simulink model "My_Nonlinear_with_controller"  (R2021b)
settings: Solver=VariableStepAuto  StartTime=0.0  StopTime=simTime  RelTol=1e-3
undefined symbols (not defined in the file): b, D, g, k, L, m, MoI, omega, p, p_dot, RPM, set_point, TakeStep, Theta
libraries: slpidlib x2
settings Model: Creator=Wojciech  LastModifiedBy=tanzc

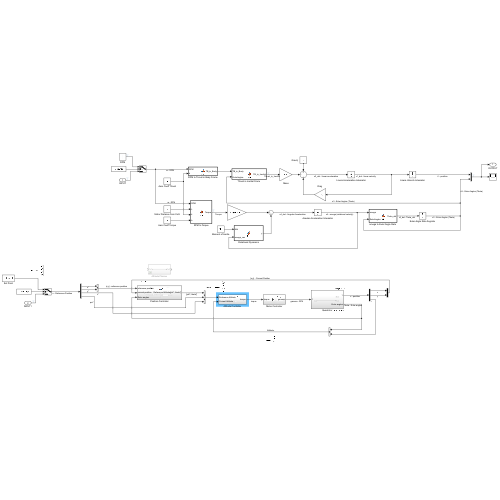
[thumbnail: Simulink's stored preview of the top-level diagram]
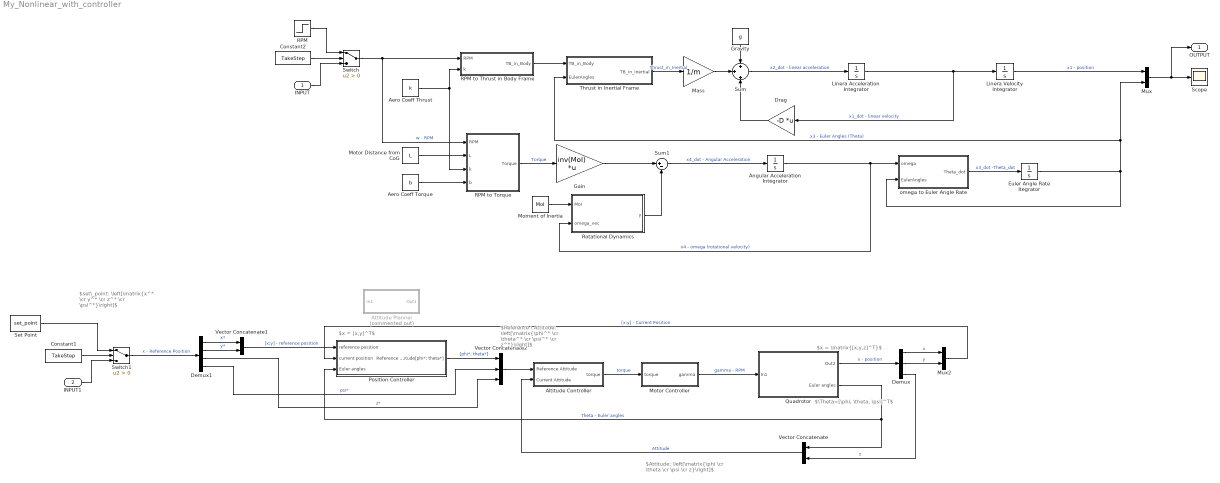
== system My_Nonlinear_with_controller ==
  note: $x = [x,y]^T$
  note: $\Theta=[\phi, \theta, \psi]^T$
  note: $x = \matrix{[x,y,z]^T}$
  note: $Attitude: \left[\matrix{\phi \cr \theta \cr \psi \cr z}\right]$
  note: $set\_point: \left[\matrix{x^* \cr y^* \cr z^* \cr \psi^*}\right]$
  note: $Reference \ Attitude: \left[\matrix{\phi^* \cr \theta^* \cr \psi^* \cr z^*}\right]$
  INPUT : Inport  PortDimensions=4
  INPUT1 : Inport  Port=2  PortDimensions=4
  Aero Coeff Thrust : Constant  Value=k
  Aero Coeff Torque : Constant  Value=b
  Altitude Controller : Subsystem
  Angular Acceleration Integrator : Integrator  Priority=4  InitialCondition=omega
  Attitude Planner : Subsystem  Commented=on
  Constant1 : Constant  Value=TakeStep
  Constant2 : Constant  Value=TakeStep
  Demux : Demux  Outputs=3
  Demux1 : Demux
  Drag : Gain  Gain=-D  Multiplication=Matrix(K*u)
  Euler Angle Rate Itegrator : Integrator  Priority=3  InitialCondition=Theta
  Gain : Gain  Gain=inv(MoI)  Multiplication=Matrix(K*u)
  Gravity : Constant  Value=g  VectorParams1D=off
  Linera Acceleration Integrator : Integrator  Priority=2  InitialCondition=p_dot
  Linera Velocity Integrator : Integrator  Priority=1  InitialCondition=p
  Mass : Gain  Gain=1/m
  Moment of Inertia : Constant  Value=MoI  VectorParams1D=off
  Motor Controller : Subsystem
  Motor Distance from CoG : Constant  Value=L
  Mux : Mux  Inputs=2
  Mux2 : Mux  Inputs=2
  Position Controller : Subsystem
  Quadrotor : Subsystem
  RPM : Step  Time=0  After=RPM  SampleTime=0
  RPM to Thrust in Body Frame : MATLAB Function  TreatAsAtomicUnit=on
  RPM to Torque : MATLAB Function  TreatAsAtomicUnit=on
  Rotational Dynamics : MATLAB Function  TreatAsAtomicUnit=on
  Scope : Scope
  Set Point : Constant  Value=set_point
  Sum : Sum  Inputs=+|+|+
  Sum1 : Sum  Inputs=|+-
  Switch : Switch  Criteria=u2 > Threshold
  Switch1 : Switch  Criteria=u2 > Threshold
  Thrust in Inertial Frame : MATLAB Function  TreatAsAtomicUnit=on
  Vector Concatenate : Concatenate
  Vector Concatenate1 : Concatenate
  Vector Concatenate2 : Concatenate  NumInputs=3
  "omega to Euler Angle Rate " : MATLAB Function  TreatAsAtomicUnit=on
  OUTPUT : Outport
  wires:
  Linera Velocity Integrator/1 -> Mux/1  "x1 - position"
  Linera Acceleration Integrator/1 -> Drag/1, Linera Velocity Integrator/1  "x1_dot - linear velocity"
  Sum/1 -> Linera Acceleration Integrator/1  "x2_dot - linear acceleration"
  Gravity/1 -> Sum/1
  RPM to Thrust in Body Frame/1(TB_in_Body) -> Thrust in Inertial Frame/1(TB_in_Body)
  Aero Coeff Thrust/1 -> RPM to Thrust in Body Frame/2(k), RPM to Torque/3(k)
  Thrust in Inertial Frame/1(TB_in_Inertial) -> Mass/1  "Thrust_in_Inertial"
  Mass/1 -> Sum/2
  Drag/1 -> Sum/3
  Motor Distance from CoG/1 -> RPM to Torque/2(L)
  Aero Coeff Torque/1 -> RPM to Torque/4(b)
  RPM to Torque/1(Torque) -> Gain/1  "Torque"
  Gain/1 -> Sum1/1
  Rotational Dynamics/1(y) -> Sum1/2
  Moment of Inertia/1 -> Rotational Dynamics/1(MoI)
  Sum1/1 -> Angular Acceleration Integrator/1  "x4_dot - Angular Acceleration"
  Angular Acceleration Integrator/1 -> "omega to Euler Angle Rate "/1(omega), Rotational Dynamics/2(omega_vec)  "x4 - omega (rotational velocity)"
  "omega to Euler Angle Rate "/1(Theta_dot) -> Euler Angle Rate Itegrator/1  "x3_dot -Theta_dot"
  Euler Angle Rate Itegrator/1 -> Mux/2, Thrust in Inertial Frame/2(EulerAngles), "omega to Euler Angle Rate "/2(EulerAngles)  "x3 - Euler Angles (Theta)"
  Mux/1 -> OUTPUT/1, Scope/1
  Constant2/1 -> Switch/2
  INPUT/1 -> Switch/3
  RPM/1 -> Switch/1
  Switch/1 -> RPM to Thrust in Body Frame/1(RPM), RPM to Torque/1(RPM)  "w - RPM"
  Quadrotor/1(Out2) -> Demux/1  "x - position"
  Quadrotor/2(Euler angles) -> Position Controller/3(Euler angles), Vector Concatenate/1  "Theta - Euler angles"
  Vector Concatenate/1 -> Altitude Controller/2(Current Attitude)  "Attitude"
  Demux/1 -> Mux2/1  "x"
  Demux/2 -> Mux2/2  "y"
  Mux2/1 -> Position Controller/2(current position)  "[x;y] - Current Position"
  Set Point/1 -> Switch1/1
  Constant1/1 -> Switch1/2
  INPUT1/1 -> Switch1/3
  Motor Controller/1(gamma) -> Quadrotor/1(In1)  "gamma - RPM"
  Altitude Controller/1(torque) -> Motor Controller/1(torque)  "torque"
  Switch1/1 -> Demux1/1  "x - Reference Position"
  Demux1/1 -> Vector Concatenate1/1  "x*"
  Demux1/2 -> Vector Concatenate1/2  "y*"
  Demux1/3 -> Vector Concatenate2/3  "z*"
  Vector Concatenate1/1 -> Position Controller/1(reference position)  "[x;y] - reference position"
  Position Controller/1(Reference Attitude[phi*; theta*]) -> Vector Concatenate2/1  "[phi*; theta*]"
  Vector Concatenate2/1 -> Altitude Controller/1(Reference Attitude)
  Demux1/4 -> Vector Concatenate2/2  "psi*"
  Demux/3 -> Vector Concatenate/2  "z"

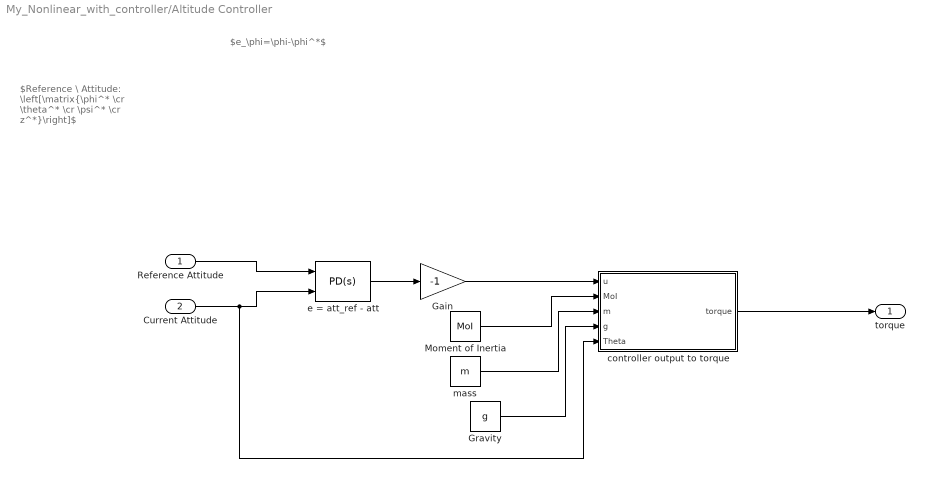
== system My_Nonlinear_with_controller/Altitude Controller ==
  note: $e_\phi=\phi-\phi^*$
  note: $Reference \ Attitude: \left[\matrix{\phi^* \cr \theta^* \cr \psi^* \cr z^*}\right]$
  Reference Attitude : Inport
  Current Attitude : Inport  Port=2
  Gain : Gain  Gain=-1
  Gravity : Constant  Value=g  VectorParams1D=off
  Moment of Inertia : Constant  Value=MoI  VectorParams1D=off
  controller output to torque : MATLAB Function  TreatAsAtomicUnit=on
  e = att_ref - att : slpidlib/PID Controller (2DOF)  Controller=PD  Form=Parallel  TimeDomain=Continuous-time  UseExternalTs=off  SampleTime=-1  IntegratorMethod=Forward Euler  FilterMethod=Forward Euler  ControllerParametersSource=internal  P=1  I=1  D=0  UseFilter=on  N=100  b=1  c=1  TunerSelectOption=Transfer Function Based (PID Tuner App)  InitialConditionSource=internal  InitialConditionForIntegrator=0  InitialConditionForFilter=0  DifferentiatorICPrevScaledInput=0  ExternalReset=none  TrackingMode=off  Kt=1  LimitOutput=off  SatLimitsSource=internal  UpperSaturationLimit=inf  LowerSaturationLimit=-inf  LinearizeAsGain=on  AntiWindupMode=none  Kb=1  POutMin=[]  POutMax=[]  IOutMin=[]  IOutMax=[]  DOutMin=[]  DOutMax=[]  NOutMin=[]  NOutMax=[]  bOutMin=[]  bOutMax=[]  cOutMin=[]  cOutMax=[]  SumOutMin=[]  SumOutMax=[]  SaturationOutMin=[]  SaturationOutMax=[]  PParamMin=[]  PParamMax=[]  IParamMin=[]  IParamMax=[]  DParamMin=[]  DParamMax=[]  NParamMin=[]  NParamMax=[]  bParamMin=[]  bParamMax=[]  cParamMin=[]  cParamMax=[]  KbParamMin=[]  KbParamMax=[]  KtParamMin=[]  KtParamMax=[]  KbOutMin=[]  KbOutMax=[]  KtOutMin=[]  KtOutMax=[]  IntegratorOutMin=[]  IntegratorOutMax=[]  FilterOutMin=[]  FilterOutMax=[]  SumI1OutMin=[]  SumI1OutMax=[]  SumI2OutMin=[]  SumI2OutMax=[]  SumI3OutMin=[]  SumI3OutMax=[]  SumI4OutMin=[]  SumI4OutMax=[]  SumDOutMin=[]  SumDOutMax=[]  Sum1OutMin=[]  Sum1OutMax=[]  Sum2OutMin=[]  Sum2OutMax=[]  Sum3OutMin=[]  Sum3OutMax=[]  DifferentiatorOutMin=[]  DifferentiatorOutMax=[]  FilterDiffOutCoefMin=[]  FilterDiffOutCoefMax=[]  ReciprocalOutMin=[]  ReciprocalOutMax=[]  SumDenOutMin=[]  SumDenOutMax=[]  SumNumOutMin=[]  SumNumOutMax=[]  DivideOutMin=[]  DivideOutMax=[]  UdiffTsProdOutMin=[]  UdiffTsProdOutMax=[]  NTsProdOutMin=[]  NTsProdOutMax=[]  UintegralTsProdOutMin=[]  UintegralTsProdOutMax=[]  UngainTsProdOutMin=[]  UngainTsProdOutMax=[]  IntegratorContinuousStateAttributes=''  IntegratorStateMustResolveToSignalObject=off  IntegratorRTWStateStorageClass=Auto  FilterContinuousStateAttributes=''  FilterStateMustResolveToSignalObject=off  FilterRTWStateStorageClass=Auto  ParallelPVariant=InternalParameters  IdealPVariant=Disabled  IVariant=Disabled  DVariant=InternalParameters  bVariant=InternalParameters  cVariant=InternalParameters  IntegratorVariant=Disabled  SatVariant=Disabled  AWVariant=Disabled  PCopyVariant=Disabled  TRVariant=Disabled  FdbkBlocksVariant=Forward  IdealPFdbkVariant=Disabled  SatFdbkVariant=Disabled  DerivativeFilterVariant=ContFilter  NVariant=InternalParameters  NCopyVariant=Disabled  FilterICVariant=InternalICsFilter  IntegratorICVariant=Disabled  ExternalResetVariant=Disabled  TRSumVariant=Passthrough  SumFdbkVariant=Disabled  SumVariant=Sum_PD  TsampFilterVariant=InternalTs  TsampNgainVariant=Passthrough  TsampIntegralVariant=Disabled_SignalSpec  ExternalSaturationOutDataTypeStr=Inherit: Same as second input
      settings: SourceProductBaseCode=SL
  mass : Constant  Value=m
  torque : Outport
  wires:
  Reference Attitude/1 -> e = att_ref - att/1
  Current Attitude/1 -> controller output to torque/5(Theta), e = att_ref - att/2
  e = att_ref - att/1 -> Gain/1
  Gain/1 -> controller output to torque/1(u)
  Moment of Inertia/1 -> controller output to torque/2(MoI)
  mass/1 -> controller output to torque/3(m)
  Gravity/1 -> controller output to torque/4(g)
  controller output to torque/1(torque) -> torque/1

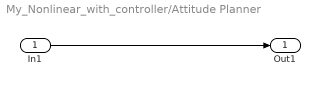
== system My_Nonlinear_with_controller/Attitude Planner ==
  In1 : Inport
  Out1 : Outport
  wires:
  In1/1 -> Out1/1

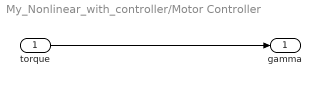
== system My_Nonlinear_with_controller/Motor Controller ==
  torque : Inport
  gamma : Outport
  wires:
  torque/1 -> gamma/1

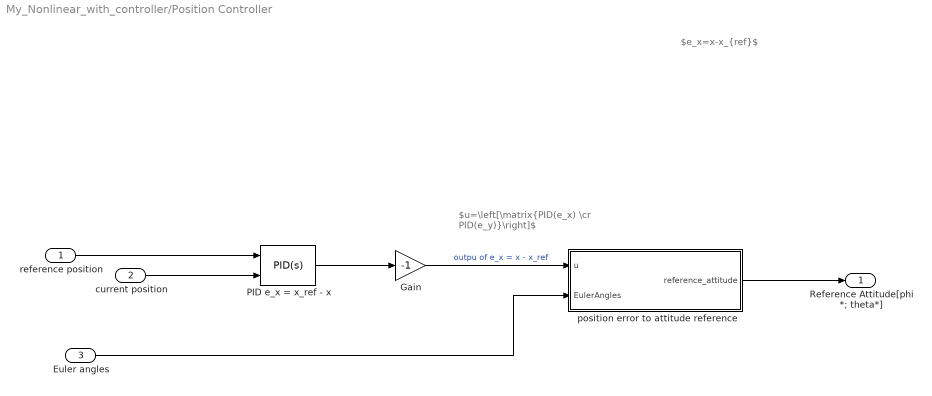
== system My_Nonlinear_with_controller/Position Controller ==
  note: $u=\left[\matrix{PID(e_x) \cr PID(e_y)}\right]$
  note: $e_x=x-x_{ref}$
  reference position : Inport
  current position : Inport  Port=2
  Euler angles : Inport  Port=3
  Gain : Gain  Gain=-1
  PID e_x = x_ref - x : slpidlib/PID Controller (2DOF)  Controller=PID  Form=Parallel  TimeDomain=Continuous-time  UseExternalTs=off  SampleTime=-1  IntegratorMethod=Forward Euler  FilterMethod=Forward Euler  ControllerParametersSource=internal  P=1  I=1  D=0  UseFilter=on  N=100  b=1  c=1  TunerSelectOption=Transfer Function Based (PID Tuner App)  InitialConditionSource=internal  InitialConditionForIntegrator=0  InitialConditionForFilter=0  DifferentiatorICPrevScaledInput=0  ExternalReset=none  TrackingMode=off  Kt=1  LimitOutput=off  SatLimitsSource=internal  UpperSaturationLimit=inf  LowerSaturationLimit=-inf  LinearizeAsGain=on  AntiWindupMode=none  Kb=1  POutMin=[]  POutMax=[]  IOutMin=[]  IOutMax=[]  DOutMin=[]  DOutMax=[]  NOutMin=[]  NOutMax=[]  bOutMin=[]  bOutMax=[]  cOutMin=[]  cOutMax=[]  SumOutMin=[]  SumOutMax=[]  SaturationOutMin=[]  SaturationOutMax=[]  PParamMin=[]  PParamMax=[]  IParamMin=[]  IParamMax=[]  DParamMin=[]  DParamMax=[]  NParamMin=[]  NParamMax=[]  bParamMin=[]  bParamMax=[]  cParamMin=[]  cParamMax=[]  KbParamMin=[]  KbParamMax=[]  KtParamMin=[]  KtParamMax=[]  KbOutMin=[]  KbOutMax=[]  KtOutMin=[]  KtOutMax=[]  IntegratorOutMin=[]  IntegratorOutMax=[]  FilterOutMin=[]  FilterOutMax=[]  SumI1OutMin=[]  SumI1OutMax=[]  SumI2OutMin=[]  SumI2OutMax=[]  SumI3OutMin=[]  SumI3OutMax=[]  SumI4OutMin=[]  SumI4OutMax=[]  SumDOutMin=[]  SumDOutMax=[]  Sum1OutMin=[]  Sum1OutMax=[]  Sum2OutMin=[]  Sum2OutMax=[]  Sum3OutMin=[]  Sum3OutMax=[]  DifferentiatorOutMin=[]  DifferentiatorOutMax=[]  FilterDiffOutCoefMin=[]  FilterDiffOutCoefMax=[]  ReciprocalOutMin=[]  ReciprocalOutMax=[]  SumDenOutMin=[]  SumDenOutMax=[]  SumNumOutMin=[]  SumNumOutMax=[]  DivideOutMin=[]  DivideOutMax=[]  UdiffTsProdOutMin=[]  UdiffTsProdOutMax=[]  NTsProdOutMin=[]  NTsProdOutMax=[]  UintegralTsProdOutMin=[]  UintegralTsProdOutMax=[]  UngainTsProdOutMin=[]  UngainTsProdOutMax=[]  IntegratorContinuousStateAttributes=''  IntegratorStateMustResolveToSignalObject=off  IntegratorRTWStateStorageClass=Auto  FilterContinuousStateAttributes=''  FilterStateMustResolveToSignalObject=off  FilterRTWStateStorageClass=Auto  ParallelPVariant=InternalParameters  IdealPVariant=Disabled  IVariant=InternalParameters  DVariant=InternalParameters  bVariant=InternalParameters  cVariant=InternalParameters  IntegratorVariant=Continuous  SatVariant=Disabled  AWVariant=Passthrough  PCopyVariant=Disabled  TRVariant=Disabled  FdbkBlocksVariant=Forward  IdealPFdbkVariant=Disabled  SatFdbkVariant=Disabled  DerivativeFilterVariant=ContFilter  NVariant=InternalParameters  NCopyVariant=Disabled  FilterICVariant=InternalICsFilter  IntegratorICVariant=InternalICs  ExternalResetVariant=Disabled  TRSumVariant=Passthrough  SumFdbkVariant=Disabled  SumVariant=Sum_PID  TsampFilterVariant=InternalTs  TsampNgainVariant=Passthrough  TsampIntegralVariant=Passthrough  ExternalSaturationOutDataTypeStr=Inherit: Same as second input
      settings: SourceProductBaseCode=SL
  position error to attitude reference : MATLAB Function  TreatAsAtomicUnit=on
  Reference Attitude[phi*; theta*] : Outport
  wires:
  PID e_x = x_ref - x/1 -> Gain/1
  reference position/1 -> PID e_x = x_ref - x/1
  current position/1 -> PID e_x = x_ref - x/2
  Gain/1 -> position error to attitude reference/1(u)  "outpu of e_x = x - x_ref"
  Euler angles/1 -> position error to attitude reference/2(EulerAngles)
  position error to attitude reference/1(reference_attitude) -> Reference Attitude[phi*; theta*]/1

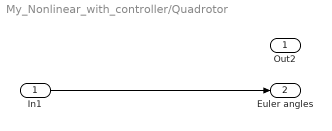
== system My_Nonlinear_with_controller/Quadrotor ==
  In1 : Inport
  Out2 : Outport
  Euler angles : Outport  Port=2
  wires:
  In1/1 -> Euler angles/1

== matlab function My_Nonlinear_with_controller/RPM to Thrust in Body Frame ==
  data: RPM input; TB_in_Body output; k input
function TB_in_Body = fcn(RPM, k)
TB_in_Body = k * [0; 0; RPM'*RPM];

== matlab function My_Nonlinear_with_controller/Thrust in Inertial Frame ==
  data: TB_in_Body input; EulerAngles input; TB_in_Inertial output
function TB_in_Inertial = fcn(TB_in_Body, EulerAngles)

phi = EulerAngles(1);
theta = EulerAngles(2);
psi = EulerAngles(3);

R = [cos(psi)*cos(theta), cos(psi)*sin(theta)*sin(phi) - sin(psi)*cos(phi), cos(psi)*sin(theta)*cos(phi) + sin(psi)*sin(phi);
    sin(psi)*cos(theta), sin(psi)*sin(theta)*sin(phi) + cos(psi)*cos(phi), sin(psi)*sin(theta)*cos(phi) - cos(psi)*sin(phi);
    -sin(theta), cos(theta)*sin(phi), cos(theta)*cos(phi)];

TB_in_Inertial = R*TB_in_Body;

== matlab function My_Nonlinear_with_controller/RPM to Torque ==
  data: RPM input; Torque output; L input; k input; b input
function Torque = fcn(RPM, L, k, b)

Torque = [  L*k*(RPM(1)^2 - RPM(3)^2); ...
            L*k*(RPM(2)^2 - RPM(4)^2); ...
            b * (RPM(1)^2 - RPM(2)^2 + RPM(3)^2 - RPM(4)^2)];

== matlab function My_Nonlinear_with_controller/Rotational Dynamics ==
  data: MoI input; omega_vec input; y output
function y = fcn(MoI, omega_vec)
Ixx = MoI(1,1);
Iyy = MoI(2,2);
Izz = MoI(3,3);

omega_x = omega_vec(1);
omega_y = omega_vec(2);
omega_z = omega_vec(3);

y = [ (Iyy-Izz)/Ixx*omega_y*omega_z; ...
      (Izz-Ixx)/Iyy*omega_x*omega_z; ...
      (Ixx-Iyy)/Izz*omega_x*omega_y];

== matlab function My_Nonlinear_with_controller/omega to Euler Angle Rate  ==
  data: omega input; Theta_dot output; EulerAngles input
function Theta_dot = fcn(omega, EulerAngles)

phi = EulerAngles(1);
theta = EulerAngles(2);
psi = EulerAngles(3);

B = [ 1, 0, -sin(theta); ...
      0, cos(phi), cos(theta)*sin(phi); ...
      0, -sin(phi), cos(theta)*cos(phi)];
  
Theta_dot = pinv(B)*omega;

== matlab function My_Nonlinear_with_controller/Position Controller/position error to attitude reference ==
  data: u input; reference_attitude output; EulerAngles input
function reference_attitude = fcn(u, EulerAngles)

% input:
% u = [PID(ex), PID(ey)]^T
% EulerAngles = [phi, theta, psi]^T

% output:
% reference_attitude = [phi*, theta*]^T

u = [u;0];
phi = EulerAngles(1);
theta = EulerAngles(2);
psi = EulerAngles(3);

rotmZYX = eul2rotm([psi, theta, phi]);


reference_attitude = [0 1 0; -1 0 0] * rotmZYX * u;

== matlab function My_Nonlinear_with_controller/Altitude Controller/controller output to torque ==
  data: u input; torque output; MoI input; m input; g input; Theta input
function torque = fcn(u, MoI, m, g, Theta)

u_phi = u(1);
u_theta = u(2);
u_psi = u(3);
F_cz = -u(4);

Ixx = MoI(1,1);
Iyy = MoI(2,2);
Izz = MoI(3,3);

phi = Theta(1);
theta = Theta(2);

torque = [  -Ixx * u_phi;
            -Iyy * u_theta;
            -Izz * u_psi;
            (m * g + F_cz)/(k * cos(phi) * cos(theta))];
